simulink model "observador_orden_reducido_accion_integral_DISCRETO"  (R2023b)
settings: Solver=VariableStepAuto  StartTime=0.0  StopTime=10.0  RelTol=1e-3
values from neighbouring files (symbols this model uses):
  J_eq = J_m + J_l/(r^2)    (= 1.97847222222e-05)    [constantes.m]    (also in test_polos_PID.m = J_m + J_l/(r^2))
  Ke_i = 3.2768e10    (= 32768000000)    [constantes.m]
  Ke_theta_2 = 9.6e3    (= 9600)    [constantes.m]
  Ke_w_2 = 3.072e7    (= 30720000)    [constantes.m]
  Ts = 2*pi/(10*5000)    (= 0.000125663706144)    [constantes.m]    (also in test_polos_PID.m = 40)
undefined symbols (not defined in the file or in its folder): DiscIntNeverNeededParam
settings Model: Creator=rodri  LastModifiedBy=Nahuel

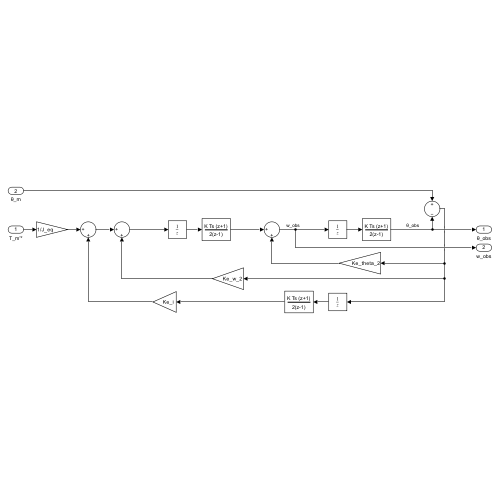
[thumbnail: Simulink's stored preview of the top-level diagram]
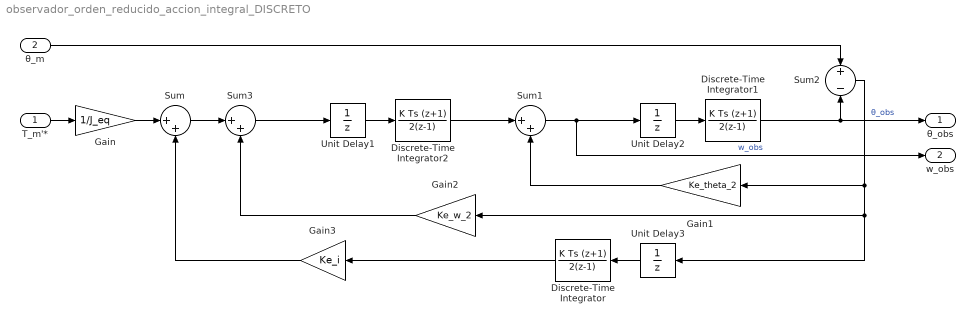
== system observador_orden_reducido_accion_integral_DISCRETO ==
  T_m'* : Inport
  θ_m : Inport  Port=2
  Discrete-Time Integrator : DiscreteIntegrator  IntegratorMethod=Integration: Trapezoidal  SampleTime=Ts  ICPrevOutput=DiscIntNeverNeededParam  ICPrevScaledInput=DiscIntNeverNeededParam
  Discrete-Time Integrator1 : DiscreteIntegrator  IntegratorMethod=Integration: Trapezoidal  SampleTime=Ts  ICPrevOutput=DiscIntNeverNeededParam  ICPrevScaledInput=DiscIntNeverNeededParam
  Discrete-Time Integrator2 : DiscreteIntegrator  IntegratorMethod=Integration: Trapezoidal  SampleTime=Ts  ICPrevOutput=DiscIntNeverNeededParam  ICPrevScaledInput=DiscIntNeverNeededParam
  Gain : Gain  Gain=1/J_eq
  Gain1 : Gain  Gain=Ke_theta_2
  Gain2 : Gain  Gain=Ke_w_2
  Gain3 : Gain  Gain=Ke_i
  Sum : Sum  Inputs=|++
  Sum1 : Sum  Inputs=|++
  Sum2 : Sum  Inputs=+-
  Sum3 : Sum  Inputs=|++
  Unit Delay1 : UnitDelay  SampleTime=Ts  HasFrameUpgradeWarning=on
  Unit Delay2 : UnitDelay  SampleTime=Ts  HasFrameUpgradeWarning=on
  Unit Delay3 : UnitDelay  SampleTime=Ts  HasFrameUpgradeWarning=on
  θ_obs : Outport
  w_obs : Outport  Port=2
  wires:
  Sum1/1 -> Unit Delay2/1, w_obs/1  "w_obs"
  θ_m/1 -> Sum2/1
  Gain2/1 -> Sum3/2
  Gain1/1 -> Sum1/2
  Sum2/1 -> Gain1/1, Unit Delay3/1, Gain2/1
  Discrete-Time Integrator2/1 -> Sum1/1
  Discrete-Time Integrator1/1 -> θ_obs/1, Sum2/2  "θ_obs"
  Sum/1 -> Sum3/1
  T_m'*/1 -> Gain/1
  Gain/1 -> Sum/1
  Discrete-Time Integrator/1 -> Gain3/1
  Gain3/1 -> Sum/2
  Sum3/1 -> Unit Delay1/1
  Unit Delay1/1 -> Discrete-Time Integrator2/1
  Unit Delay2/1 -> Discrete-Time Integrator1/1
  Unit Delay3/1 -> Discrete-Time Integrator/1
